simulink model "PID_Controller"  (R2020b)
settings: Solver=ode45  StartTime=0.0  StopTime=0.08  RelTol=1e-3
PostLoadFcn:
  | J=3.2284e-6;
  | b=3.5077e-6;
  | K=0.0274;
  | R=4;
  | L=2.75e-6;
  | 
  | Kp=40.6275;
  | Ki=331.2128;
  | Kd=0.4934;
InitFcn:
  | J=3.2284e-6;
  | b=3.5077e-6;
  | K=0.0274;
  | R=4;
  | L=2.75e-6;
  | 
  | Kp=40.6275;
  | Ki=331.2128;
  | Kd=0.4934;
settings Model: Creator=home  LastModifiedBy=home
settings DataIOCC: SaveOutput=off  SaveTime=off

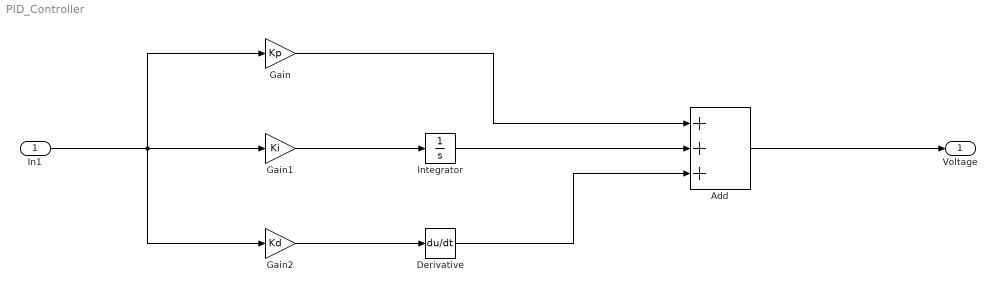
== system PID_Controller ==
  In1 : Inport  OutDataTypeStr=double  PortDimensions=1  SampleTime=0
  Add : Sum  Inputs=+++
  Derivative : Derivative
  Gain : Gain  Gain=Kp
  Gain1 : Gain  Gain=Ki
  Gain2 : Gain  Gain=Kd
  Integrator : Integrator
  Voltage : Outport  OutDataTypeStr=double  PortDimensions=1  SampleTime=0
  wires:
  Gain1/1 -> Integrator/1
  Gain2/1 -> Derivative/1
  Integrator/1 -> Add/2
  Gain/1 -> Add/1
  Derivative/1 -> Add/3
  Add/1 -> Voltage/1
  In1/1 -> Gain1/1, Gain/1, Gain2/1
